simulink model "control_project3"  (R2015a)
settings: Solver=ode45  StartTime=0.0  StopTime=10.0  RelTol=1e-3
libraries: simulink x2
settings Model: Creator=Farhan Fuad  LastModifiedBy=Farhan Fuad

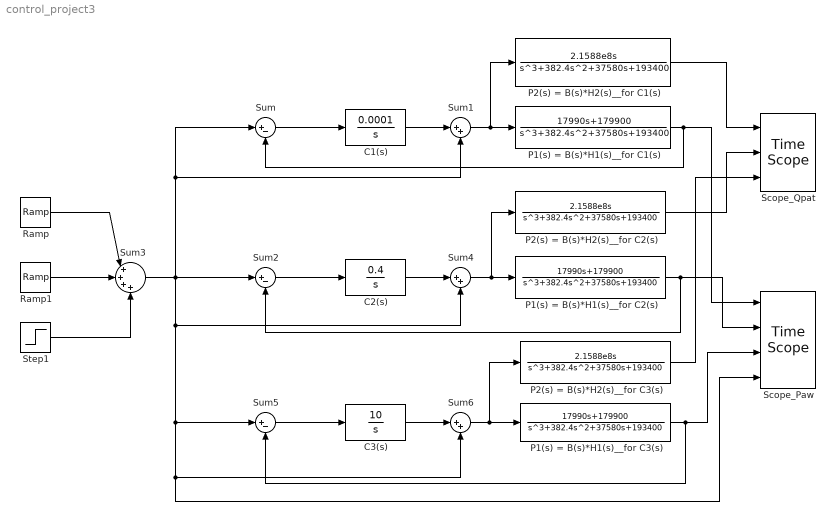
== system control_project3 ==
  C1(s) : TransferFcn  Numerator=[0 0.0001]  Denominator=[1 0]
  C2(s) : TransferFcn  Numerator=[0 0.4]  Denominator=[1 0]
  C3(s) : TransferFcn  Numerator=[0 10]  Denominator=[1 0]
  P1(s) = B(s)*H1(s)__for C1(s) : TransferFcn  Numerator=[0 0 17990 179900]  Denominator=[1 382.4 37580 193400]
  P1(s) = B(s)*H1(s)__for C2(s) : TransferFcn  Numerator=[0 0 17990 179900]  Denominator=[1 382.4 37580 193400]
  P1(s) = B(s)*H1(s)__for C3(s) : TransferFcn  Numerator=[0 0 17990 179900]  Denominator=[1 382.4 37580 193400]
  P2(s) = B(s)*H2(s)__for C1(s) : TransferFcn  Numerator=[0 0 2.1588e8 0]  Denominator=[1 382.4 37580 193400]
  P2(s) = B(s)*H2(s)__for C2(s) : TransferFcn  Numerator=[0 0 2.1588e8 0]  Denominator=[1 382.4 37580 193400]
  P2(s) = B(s)*H2(s)__for C3(s) : TransferFcn  Numerator=[0 0 2.1588e8 0]  Denominator=[1 382.4 37580 193400]
  Ramp : simulink/Sources/Ramp  slope=64.865  start=1  X0=0
  Ramp1 : simulink/Sources/Ramp  slope=-64.865  start=1.23125  X0=0
  Scope_Paw : TimeScope  NumInputPorts=4
  Scope_Qpat : TimeScope  NumInputPorts=3
  Step1 : Step  Time=5  After=-15  SampleTime=0
  Sum : Sum  Inputs=|+-
  Sum1 : Sum  Inputs=|++
  Sum2 : Sum  Inputs=|+-
  Sum3 : Sum  Inputs=|++++
  Sum4 : Sum  Inputs=|++
  Sum5 : Sum  Inputs=|+-
  Sum6 : Sum  Inputs=|++
  wires:
  Ramp/1 -> Sum3/1
  Ramp1/1 -> Sum3/2
  Step1/1 -> Sum3/4
  Sum/1 -> C1(s)/1
  C1(s)/1 -> Sum1/1
  Sum2/1 -> C2(s)/1
  C2(s)/1 -> Sum4/1
  Sum5/1 -> C3(s)/1
  C3(s)/1 -> Sum6/1
  P2(s) = B(s)*H2(s)__for C1(s)/1 -> Scope_Qpat/1
  P2(s) = B(s)*H2(s)__for C2(s)/1 -> Scope_Qpat/2
  P2(s) = B(s)*H2(s)__for C3(s)/1 -> Scope_Qpat/3
  P1(s) = B(s)*H1(s)__for C1(s)/1 -> Scope_Paw/1, Sum/2
  P1(s) = B(s)*H1(s)__for C2(s)/1 -> Scope_Paw/2, Sum2/2
  P1(s) = B(s)*H1(s)__for C3(s)/1 -> Scope_Paw/3, Sum5/2
  Sum3/1 -> Sum4/2, Sum5/1, Scope_Paw/4, Sum6/2, Sum2/1, Sum1/2, Sum/1
  Sum1/1 -> P1(s) = B(s)*H1(s)__for C1(s)/1, P2(s) = B(s)*H2(s)__for C1(s)/1
  Sum4/1 -> P1(s) = B(s)*H1(s)__for C2(s)/1, P2(s) = B(s)*H2(s)__for C2(s)/1
  Sum6/1 -> P1(s) = B(s)*H1(s)__for C3(s)/1, P2(s) = B(s)*H2(s)__for C3(s)/1
